simulink model "untitled"  (Simulink 7.6)
settings: Solver=ode4  StartTime=0.0  StopTime=inf  FixedStep=1  RelTol=1e-3
settings Model: Creator=Tao  LastModifiedBy=Tao

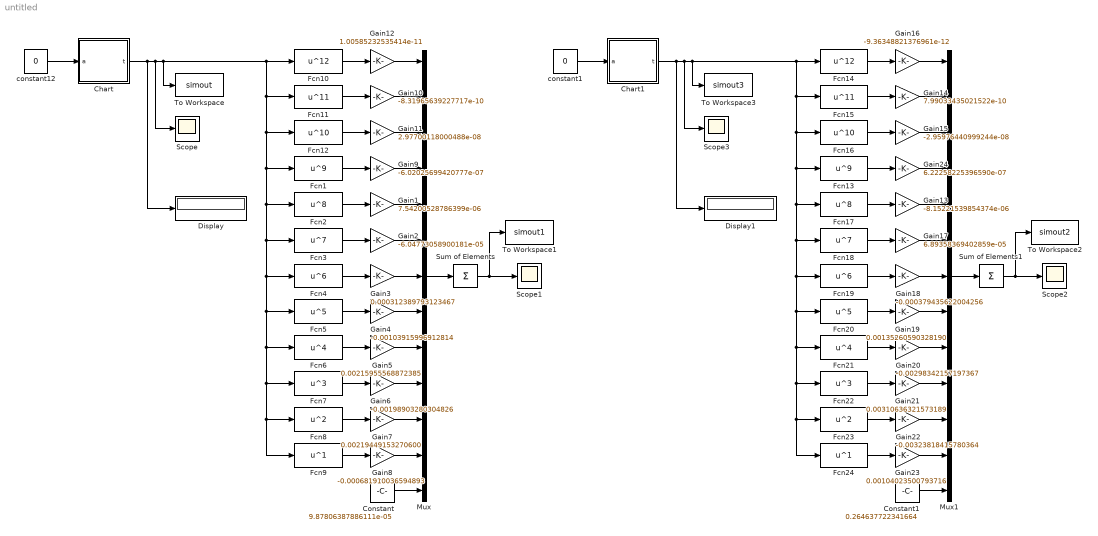
== system untitled ==
  Chart : Stateflow chart  TreatAsAtomicUnit=on
  Chart1 : Stateflow chart  TreatAsAtomicUnit=on
  Constant : Constant  Value=9.87806387886111e-05
  Constant1 : Constant  Value=0.264637722341664
  Display : Display
  Display1 : Display
  Fcn1 : Fcn  Expr=u^9
  Fcn10 : Fcn  Expr=u^12
  Fcn11 : Fcn  Expr=u^11
  Fcn12 : Fcn  Expr=u^10
  Fcn13 : Fcn  Expr=u^9
  Fcn14 : Fcn  Expr=u^12
  Fcn15 : Fcn  Expr=u^11
  Fcn16 : Fcn  Expr=u^10
  Fcn17 : Fcn  Expr=u^8
  Fcn18 : Fcn  Expr=u^7
  Fcn19 : Fcn  Expr=u^6
  Fcn2 : Fcn  Expr=u^8
  Fcn20 : Fcn  Expr=u^5
  Fcn21 : Fcn  Expr=u^4
  Fcn22 : Fcn  Expr=u^3
  Fcn23 : Fcn  Expr=u^2
  Fcn24 : Fcn  Expr=u^1
  Fcn3 : Fcn  Expr=u^7
  Fcn4 : Fcn  Expr=u^6
  Fcn5 : Fcn  Expr=u^5
  Fcn6 : Fcn  Expr=u^4
  Fcn7 : Fcn  Expr=u^3
  Fcn8 : Fcn  Expr=u^2
  Fcn9 : Fcn  Expr=u^1
  Gain1 : Gain  Gain=7.54200528786399e-06
  Gain10 : Gain  Gain=-8.31965639227717e-10
  Gain11 : Gain  Gain=2.97700118000488e-08
  Gain12 : Gain  Gain=1.00585232535414e-11
  Gain13 : Gain  Gain=-8.15221539854374e-06
  Gain14 : Gain  Gain=7.99033435021522e-10
  Gain15 : Gain  Gain=-2.95976440999244e-08
  Gain16 : Gain  Gain=-9.36348821376961e-12
  Gain17 : Gain  Gain=6.89358369402859e-05
  Gain18 : Gain  Gain=-0.000379435622004256
  Gain19 : Gain  Gain=0.00135260590328190
  Gain2 : Gain  Gain=-6.04773058900181e-05
  Gain20 : Gain  Gain=-0.00298342157197367
  Gain21 : Gain  Gain=0.00310636321573189
  Gain22 : Gain  Gain=-0.00323818415780364
  Gain23 : Gain  Gain=0.00104023500793716
  Gain24 : Gain  Gain=6.22258225396590e-07
  Gain3 : Gain  Gain=0.000312389793123467
  Gain4 : Gain  Gain=-0.00103915996912814
  Gain5 : Gain  Gain=0.00215955568872385
  Gain6 : Gain  Gain=-0.00198903280304826
  Gain7 : Gain  Gain=0.00219449153270600
  Gain8 : Gain  Gain=-0.000681910036594893
  Gain9 : Gain  Gain=-6.02025699420777e-07
  Mux : Mux  Inputs=13
  Mux1 : Mux  Inputs=13
  Scope{,1..3} (4 alike) : Scope
      Scope settings: YMin=12.52  YMax=12.555
      Scope2 settings: SaveName=ScopeData2
      Scope3 settings: YMin=12.52  YMax=12.555  SaveName=ScopeData3
  Sum of Elements : Sum  Inputs=+
  Sum of Elements1 : Sum  Inputs=+
  To Workspace : ToWorkspace  VariableName=simout  SampleTime=-1  SaveFormat=Structure
  To Workspace1 : ToWorkspace  VariableName=simout1  SampleTime=-1  SaveFormat=Structure
  To Workspace2 : ToWorkspace  VariableName=simout2  SampleTime=-1  SaveFormat=Structure
  To Workspace3 : ToWorkspace  VariableName=simout3  SampleTime=-1  SaveFormat=Structure
  constant1 : Constant  Value=0
      settings: OpenFcn=|
      | if get_param(gcb,'value')=='1',
      | set_param(gcb,'value','0');
      | else
      | set_param(gcb,'value','1');end
  constant12 : Constant  Value=0
      settings: OpenFcn=|
      | if get_param(gcb,'value')=='1',
      | set_param(gcb,'value','0');
      | else
      | set_param(gcb,'value','1');end
  wires:
  constant12/1 -> Chart/1(a)
  Chart/1(t) -> Display/1, Scope/1, To Workspace/1, Fcn10/1, Fcn11/1, Fcn12/1, Fcn1/1, Fcn2/1, Fcn3/1, Fcn4/1, Fcn5/1, Fcn6/1, Fcn7/1, Fcn9/1, Fcn8/1
  Fcn2/1 -> Gain1/1
  Fcn3/1 -> Gain2/1
  Fcn4/1 -> Gain3/1
  Fcn5/1 -> Gain4/1
  Fcn6/1 -> Gain5/1
  Fcn7/1 -> Gain6/1
  Fcn8/1 -> Gain7/1
  Fcn1/1 -> Gain9/1
  Gain9/1 -> Mux/4
  Gain1/1 -> Mux/5
  Gain2/1 -> Mux/6
  Gain3/1 -> Mux/7
  Gain4/1 -> Mux/8
  Gain5/1 -> Mux/9
  Gain6/1 -> Mux/10
  Gain7/1 -> Mux/11
  Constant/1 -> Mux/13
  Mux/1 -> Sum of Elements/1
  Sum of Elements/1 -> Scope1/1, To Workspace1/1
  Fcn9/1 -> Gain8/1
  Gain8/1 -> Mux/12
  Fcn11/1 -> Gain10/1
  Fcn12/1 -> Gain11/1
  Fcn10/1 -> Gain12/1
  Gain12/1 -> Mux/1
  Gain10/1 -> Mux/2
  Gain11/1 -> Mux/3
  Fcn17/1 -> Gain13/1
  Fcn18/1 -> Gain17/1
  Fcn19/1 -> Gain18/1
  Fcn20/1 -> Gain19/1
  Fcn21/1 -> Gain20/1
  Fcn22/1 -> Gain21/1
  Fcn23/1 -> Gain22/1
  Fcn13/1 -> Gain24/1
  Gain24/1 -> Mux1/4
  Gain13/1 -> Mux1/5
  Gain17/1 -> Mux1/6
  Gain18/1 -> Mux1/7
  Gain19/1 -> Mux1/8
  Gain20/1 -> Mux1/9
  Gain21/1 -> Mux1/10
  Gain22/1 -> Mux1/11
  Constant1/1 -> Mux1/13
  Mux1/1 -> Sum of Elements1/1
  Sum of Elements1/1 -> To Workspace2/1, Scope2/1
  Fcn24/1 -> Gain23/1
  Gain23/1 -> Mux1/12
  Fcn15/1 -> Gain14/1
  Fcn16/1 -> Gain15/1
  Fcn14/1 -> Gain16/1
  Gain16/1 -> Mux1/1
  Gain14/1 -> Mux1/2
  Gain15/1 -> Mux1/3
  constant1/1 -> Chart1/1(a)
  Chart1/1(t) -> Fcn23/1, Fcn24/1, Fcn22/1, Fcn21/1, Fcn20/1, Fcn19/1, Fcn18/1, Fcn17/1, Fcn13/1, Fcn16/1, Fcn15/1, Fcn14/1, To Workspace3/1, Scope3/1, Display1/1

== stateflow chart Chart ==
  state on1
    en:
    x=0;
    t=0;
  state on2
    entry:
    x++;
    t=x*0.002
  (default) -> on1
  on1 -> on2 : [a==1]
  (junction 5) -> on1 [order 2] : [a==0]
  on2 -> (junction 5)
  (junction 5) -> on2 [order 1] : [a==1]
  data: a input double; x local double; t output double

== stateflow chart Chart1 ==
  state on1
    en:
    x=0;
    t=0;
  state on2
    entry:
    x++;
    t=x*0.002
  (default) -> on1
  on1 -> on2 : [a==1]
  (junction 18) -> on1 [order 2] : [a==0]
  on2 -> (junction 18)
  (junction 18) -> on2 [order 1] : [a==1]
  data: a input double; x local double; t output double
